simulink model "spm_sim"  (R2024b)
settings: Solver=VariableStepAuto  StartTime=0.0  StopTime=3  RelTol=1e-3
libraries: simulink x7
settings Model: Creator=odurh  LastModifiedBy=odurh
settings RTWCC: GPUComputeCapability=3.5

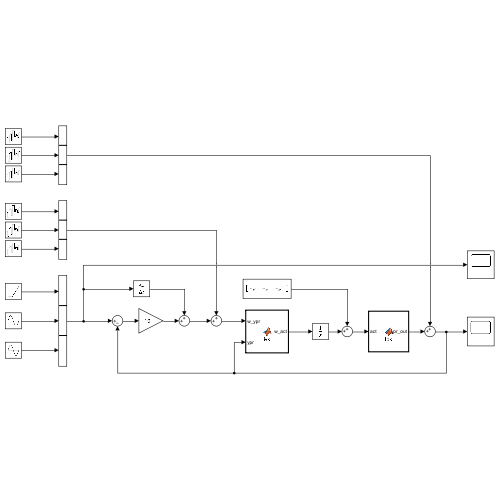
[thumbnail: Simulink's stored preview of the top-level diagram]
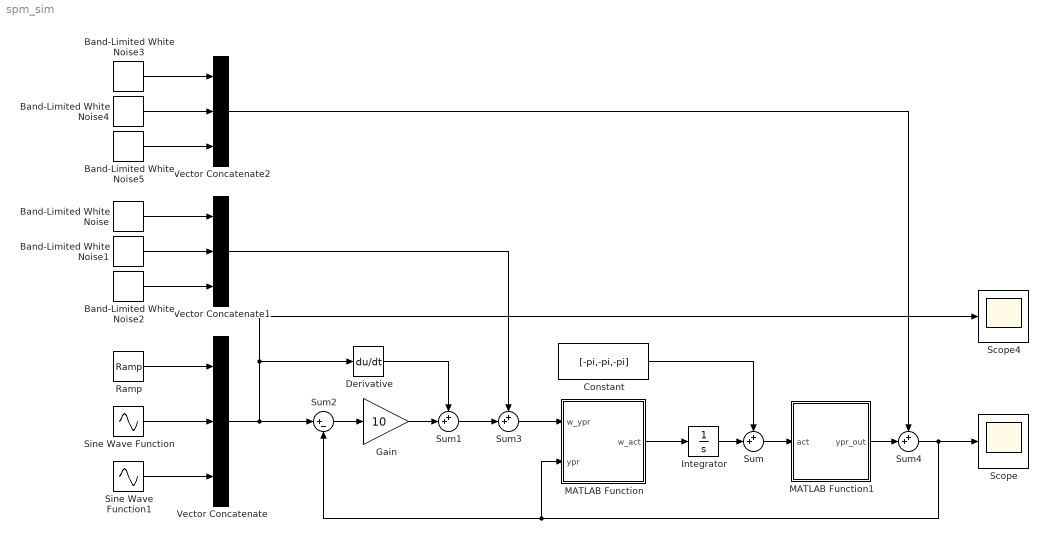
== system spm_sim ==
  Band-Limited White Noise : simulink/Sources/Band-Limited White Noise  Cov=[0.05]  Ts=1  seed=[23341]
  Band-Limited White Noise1 : simulink/Sources/Band-Limited White Noise  Cov=[0.05]  Ts=1  seed=[23342]
  Band-Limited White Noise2 : simulink/Sources/Band-Limited White Noise  Cov=[0.05]  Ts=1  seed=[23343]
  Band-Limited White Noise3 : simulink/Sources/Band-Limited White Noise  Cov=[0.005]  Ts=0.5  seed=[23346]
  Band-Limited White Noise4 : simulink/Sources/Band-Limited White Noise  Cov=[0.005]  Ts=0.5  seed=[23345]
  Band-Limited White Noise5 : simulink/Sources/Band-Limited White Noise  Cov=[0.005]  Ts=0.5  seed=[23344]
  Constant : Constant  Value=[-pi,-pi,-pi]
  Derivative : Derivative
  Gain : Gain  Gain=10
  Integrator : Integrator
  MATLAB Function : MATLAB Function  TreatAsAtomicUnit=on
  MATLAB Function1 : MATLAB Function  TreatAsAtomicUnit=on
  Ramp : simulink/Sources/Ramp  slope=1  start=0  InitialOutput=-pi
  Scope : Scope
  Scope4 : Scope
  Sine Wave Function : Sin  Amplitude=0.25  Frequency=2  SampleTime=0
  Sine Wave Function1 : Sin  Amplitude=-0.25  Frequency=2  SampleTime=0
  Sum{,1,3..4} (4 alike) : Sum  Inputs=++|
  Sum2 : Sum  Inputs=|+-
  Vector Concatenate : Concatenate  NumInputs=3
  Vector Concatenate1 : Concatenate  NumInputs=3
  Vector Concatenate2 : Concatenate  NumInputs=3
  wires:
  Ramp/1 -> Vector Concatenate/1
  Sine Wave Function/1 -> Vector Concatenate/2
  Sine Wave Function1/1 -> Vector Concatenate/3
  MATLAB Function/1(w_act) -> Integrator/1
  Vector Concatenate/1 -> Sum2/1, Scope4/1, Derivative/1
  Sum/1 -> MATLAB Function1/1(act)
  Gain/1 -> Sum1/2
  Derivative/1 -> Sum1/1
  Constant/1 -> Sum/1
  Integrator/1 -> Sum/2
  Sum2/1 -> Gain/1
  Sum1/1 -> Sum3/2
  Sum3/1 -> MATLAB Function/1(w_ypr)
  Band-Limited White Noise/1 -> Vector Concatenate1/1
  Band-Limited White Noise1/1 -> Vector Concatenate1/2
  Band-Limited White Noise2/1 -> Vector Concatenate1/3
  Band-Limited White Noise4/1 -> Vector Concatenate2/2
  Band-Limited White Noise3/1 -> Vector Concatenate2/1
  Band-Limited White Noise5/1 -> Vector Concatenate2/3
  MATLAB Function1/1(ypr_out) -> Sum4/2
  Sum4/1 -> MATLAB Function/2(ypr), Sum2/2, Scope/1
  Vector Concatenate2/1 -> Sum4/1
  Vector Concatenate1/1 -> Sum3/1

== matlab function spm_sim/MATLAB Function ==
  data: w_ypr input; w_act output; ypr input
function w_act = ivk(w_ypr, ypr)
    a1 = pi/4; % alpha 1
    a2 = pi/2; % alpha 2
    b = pi/2; % beta
    
    spm = coax_spm(a1,a2,b);
    w_act = solve_ivk(spm, ypr, w_ypr);
end

== matlab function spm_sim/MATLAB Function1 ==
  data: act input; ypr_out output
function ypr_out = fpk(act)
    a1 = pi/4; % alpha 1
    a2 = pi/2; % alpha 2
    b = pi/2; % beta
    
    spm = coax_spm(a1,a2,b);
    input_angles = act + spm.actuator_origin;
    ypr_out = solve_fpk(spm, input_angles.').';
end
